simulink model "Czeta"  (R2019b)
settings: Solver=FixedStepAuto  StartTime=0.0  StopTime=10.0  FixedStep=Simulation_Step  RelTol=1e-3
undefined symbols (not defined in the file): DiscIntNeverNeededParam
settings Model: Creator=r720r  LastModifiedBy=r720r

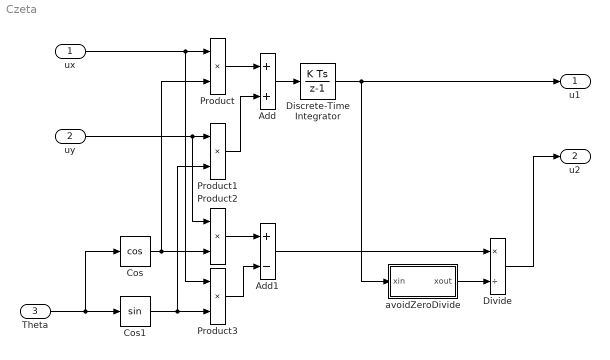
== system Czeta ==
  ux : Inport  OutDataTypeStr=double  PortDimensions=1
  uy : Inport  Port=2  OutDataTypeStr=double  PortDimensions=1
  Theta : Inport  Port=3  OutDataTypeStr=double  PortDimensions=1
  Add : Sum
  Add1 : Sum  Inputs=+-
  Cos : Trigonometry  Operator=cos
  Cos1 : Trigonometry
  Discrete-Time Integrator : DiscreteIntegrator  InitialCondition=0.001  SampleTime=-1  ICPrevOutput=DiscIntNeverNeededParam  ICPrevScaledInput=DiscIntNeverNeededParam
  Divide : Product  Inputs=*/
  Product{,1..3} (4 alike) : Product
  avoidZeroDivide : Subsystem
  u1 : Outport  OutDataTypeStr=double  PortDimensions=1
  u2 : Outport  Port=2  OutDataTypeStr=double  PortDimensions=1
  wires:
  uy/1 -> Product2/1, Product1/1
  ux/1 -> Product/1, Product3/1
  Cos/1 -> Product/2, Product2/2
  Theta/1 -> Cos1/1, Cos/1
  Cos1/1 -> Product1/2, Product3/2
  Product/1 -> Add/1
  Product1/1 -> Add/2
  Add/1 -> Discrete-Time Integrator/1
  Discrete-Time Integrator/1 -> avoidZeroDivide/1(xin), u1/1
  Product2/1 -> Add1/1
  Product3/1 -> Add1/2
  Add1/1 -> Divide/1
  avoidZeroDivide/1(xout) -> Divide/2
  Divide/1 -> u2/1

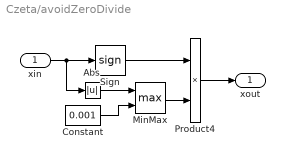
== system Czeta/avoidZeroDivide ==
  xin : Inport
  Abs : Abs
  Constant : Constant  Value=0.001
  MinMax : MinMax  Function=max  Inputs=2
  Product4 : Product
  Sign : Signum
  xout : Outport
  wires:
  Sign/1 -> Product4/1
  Abs/1 -> MinMax/1
  MinMax/1 -> Product4/2
  xin/1 -> Sign/1, Abs/1
  Constant/1 -> MinMax/2
  Product4/1 -> xout/1
